simulink model "Controll_RigidBody_R2021b"  (R2021b)
settings: Solver=ode4  StartTime=0.0  StopTime=inf  FixedStep=0.01  MaxStep=0.2  RelTol=1e-3
values from neighbouring files (symbols this model uses):
  Km1 = Km_gain    (= 0.1)    [param_EiH_VFC.m]
  Km2 = Km_gain    (= 0.1)    [param_EiH_VFC.m]
  Km3 = Km_gain    (= 0.1)    [param_EiH_VFC.m]
  Km4 = Km_gain    (= 0.1)    [param_EiH_VFC.m]
  Km5 = Km_gain    (= 0.1)    [param_EiH_VFC.m]
  Km6 = Km_gain    (= 0.1)    [param_EiH_VFC.m]
  R_threshold = 1e-8    (= 1e-08)    [param_EiH_VFC.m]
  zeta_threshold = 1e-8    (= 1e-08)    [param_EiH_VFC.m]
undefined symbols (not defined in the file or in its folder): magnitude, pzeta_d
libraries: dspnetwork x2, dspmtrx3 x1
(part 2 of 2)

== system Controll_RigidBody_R2021b/make pwm Rwm/make_Rd/3x1 -> 2norm ==
  3x1 : Inport
  Demux : Demux  Outputs=3
      settings: DisplayOption=none
  Math Function : Math  Operator=magnitude^2  SignedPower=on  SaturateOnIntegerOverflow=on
  Math Function1 : Math  Operator=sqrt  SignedPower=on  SaturateOnIntegerOverflow=on
  Sum : Sum  Inputs=+++  InputSameDT=on  SaturateOnIntegerOverflow=on  OutDataTypeStr=Inherit: Same as first input
  2 norm : Outport  VectorParamsAs1DForOutWhenUnconnected=off
  wires:
  Math Function/1 -> Demux/1
  Demux/3 -> Sum/3
  Demux/2 -> Sum/2
  Demux/1 -> Sum/1
  Sum/1 -> Math Function1/1
  Math Function1/1 -> 2 norm/1
  3x1/1 -> Math Function/1

== system Controll_RigidBody_R2021b/make pwm Rwm/make_Rd/wedge ==
  "[3x1]" : Inport
  Product1 : Product  InputSameDT=on  SaturateOnIntegerOverflow=on  OutDataTypeStr=Inherit: Same as first input
  Product2 : Product  InputSameDT=on  SaturateOnIntegerOverflow=on  OutDataTypeStr=Inherit: Same as first input
  Product3 : Product  InputSameDT=on  SaturateOnIntegerOverflow=on  OutDataTypeStr=Inherit: Same as first input
  Sum : Sum  Inputs=+++  InputSameDT=on  SaturateOnIntegerOverflow=on  OutDataTypeStr=Inherit: Same as first input
  Xaxis : Constant  Value=[0 0 0;0 0 -1;0 1 0]  VectorParams1D=off
  Yaxis : Constant  Value=[0 0 1;0 0 0;-1 0 0]  VectorParams1D=off
  Zaxis : Constant  Value=[0 -1 0;1 0 0;0 0 0]  VectorParams1D=off
  x : Gain  Gain=[1 0 0]  Multiplication=Matrix(K*u)  SaturateOnIntegerOverflow=on  OutDataTypeStr=Inherit: Same as input  ParamDataTypeStr=Inherit: Same as input
  y : Gain  Gain=[0 1 0]  Multiplication=Matrix(K*u)  SaturateOnIntegerOverflow=on  OutDataTypeStr=Inherit: Same as input  ParamDataTypeStr=Inherit: Same as input
  z : Gain  Gain=[0 0 1]  Multiplication=Matrix(K*u)  SaturateOnIntegerOverflow=on  OutDataTypeStr=Inherit: Same as input  ParamDataTypeStr=Inherit: Same as input
  "[3x3]" : Outport  VectorParamsAs1DForOutWhenUnconnected=off
  wires:
  Sum/1 -> "[3x3]"/1
  Product1/1 -> Sum/3
  Product2/1 -> Sum/1
  Product3/1 -> Sum/2
  "[3x1]"/1 -> z/1, x/1, y/1
  y/1 -> Product3/1
  Yaxis/1 -> Product3/2
  x/1 -> Product2/1
  Xaxis/1 -> Product2/2
  z/1 -> Product1/1
  Zaxis/1 -> Product1/2

== system Controll_RigidBody_R2021b/make pwm Rwm/make_Rd/zero check R_threshold ==
  In1 : Inport
  Switch : Switch  Threshold=R_threshold  SaturateOnIntegerOverflow=on  InputSameDT=on
  norm_xi : Constant  Value=R_threshold  VectorParams1D=off
  Out1 : Outport  VectorParamsAs1DForOutWhenUnconnected=off
  wires:
  Switch/1 -> Out1/1
  In1/1 -> Switch/2, Switch/1
  norm_xi/1 -> Switch/3

== matlab function Controll_RigidBody_R2021b/make Vwm/MATLAB Function ==
  data: Ad_ge input; inv_Ad_ge output
function inv_Ad_ge = fcn(Ad_ge)

inv_Ad_ge = inv(Ad_ge);
